simulink model "power_SVPWM_3Level"  (R2022a)
settings: Solver=FixedStepDiscrete  StartTime=0.0  StopTime=0.35  RelTol=1e-4  EnableMultiTasking=on
PreLoadFcn:
  | Ts=5e-6;          % Sample time (s)
StartFcn:
  | tic
StopFcn:
  | toc
undefined symbols (not defined in the file): D1, Delta, Lstat
libraries: spsSeriesRLCBranchLib x9, spsThreePhaseVIMeasurementLib x3, spsVoltageMeasurementLib x2, spsThreePhaseSourceLib x1, spsCurrentMeasurementLib x1, spsDCVoltageSourceLib x1, spsPower3phInstantaneousLib x1, spsSVPWMGenerator3LevelLib x1, spsIdealSwitchLib x1, spsThreeLevelNPCConverterLib x1, spsThreePhaseTransformerTwoWindingsLib x1, spspowerguiLib x1
settings Model: Creator=The MathWorks, Inc.  LastModifiedBy=jicai
settings SolverCC: AlgebraicLoopSolver=TrustRegion
settings DataIOCC: SaveFormat=Array  SaveOutput=off  SignalLogging=off  DSMLogging=off  SaveTime=off  ReturnWorkspaceOutputs=off
settings OptimizationCC: ExpressionDepthLimit=2147483647  LifeSpan=inf
settings DebuggingCC: UnderspecifiedInitializationDetection=Classic  MergeDetectMultiDrivingBlocksExec=none  SolverPrmCheckMsg=warning  SingleTaskRateTransMsg=warning  UnconnectedInputMsg=warning  UnconnectedOutputMsg=warning  UnconnectedLineMsg=warning  StateNameClashWarn=warning  SFUnexpectedBacktrackingDiag=warning  SFNoUnconditionalDefaultTransitionDiag=warning  SFExecutionAtInitializationDiag=none  SFMachineParentedDataDiag=warning  ArithmeticOperatorsInVariantConditions=warning
settings HardwareCC: ProdBitPerPointer=32  ProdBitPerSizeT=32  ProdBitPerPtrDiffT=32  ProdLargestAtomicFloat=None  ProdIntDivRoundTo=Undefined  ProdEndianess=Unspecified  ProdWordSize=32  ProdHWDeviceType=32-bit Generic
settings ModelReferenceCC: PropagateSignalLabelsOutOfModel=off
settings SFSimCC: SimUseLocalCustomCode=off  CustomCodeUndefinedFunction=UseInterfaceOnly
settings RTWCC: RTWUseLocalCustomCode=off
settings CodeAppCC: StateflowObjectComments=on
settings GRTTargetCC: TargetLangStandard=C89/C90 (ANSI)
settings ConfigComp: CovMetricSettings=dw  CovSaveCumulativeToWorkspaceVar=on  CovSaveSingleToWorkspaceVar=on  CovExternalEMLEnable=off
settings SimscapeCC: SimscapeNormalizeSystem=off

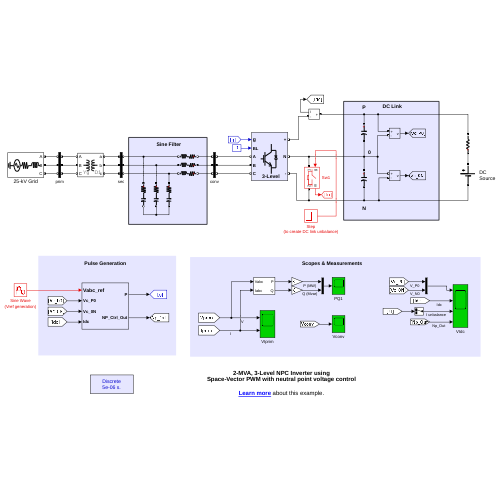
[thumbnail: Simulink's stored preview of the top-level diagram]
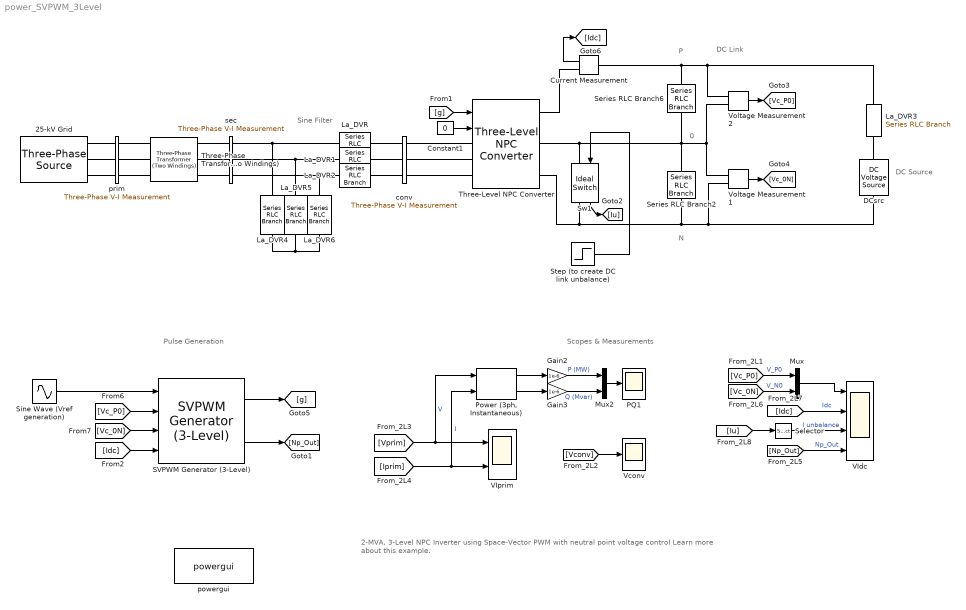
== system power_SVPWM_3Level ==
  note: DC
      | Source
  note: Scopes & Measurements
  note: 0
  note: 2-MVA, 3-Level NPC Inverter using
      | Space-Vector PWM with neutral point voltage control
      |
      | Learn more about this example.
  note: P
  note: N
  note: Sine Filter
  note: DC Link
  note: Pulse Generation
  25-kV Grid : spsThreePhaseSourceLib/Three-Phase Source  InternalConnection=Yg  VoltagePhases=off  Voltage=25e3  PhaseAngle=0  Voltage_phases=[25e3 25e3 25e3]/sqrt(3)  PhaseAngles_phases=[0 -120 +120]  Frequency=60  NonIdealSource=on  SpecifyImpedance=on  Resistance=0.8929  Inductance=16.58e-3  ShortCircuitLevel=200e6  BaseVoltage=25e3  XRratio=7  BusType=swing  Pref=10e3  Qref=0  Prefabc=[10e3, 10e3, 10e3]  Qrefabc=[0, 0, 0]  Qmin=-inf  Qmax=inf
  Constant1 : Constant  Value=0
  Current Measurement : spsCurrentMeasurementLib/Current Measurement  PhasorSimulation=off  OutputType=Complex  PSBequivalent=0
  DCsrc : spsDCVoltageSourceLib/DC Voltage Source  Amplitude=2400  Measurements=None
  Gain2 : Gain  Gain=1e-6
  Gain3 : Gain  Gain=1e-6
  La_DVR : spsSeriesRLCBranchLib/Series RLC Branch  LConnTagsString=__new0  RConnTagsString=__new0  BranchType=RL  Resistance=5e-3  Inductance=500e-6  SetiL0=off  InitialCurrent=0  Capacitance=1.0  Setx0=off  InitialVoltage=0  Measurements=None
  La_DVR1 : spsSeriesRLCBranchLib/Series RLC Branch  LConnTagsString=__new0  RConnTagsString=__new0  BranchType=RL  Resistance=5e-3  Inductance=500e-6  SetiL0=off  InitialCurrent=0  Capacitance=1.0  Setx0=off  InitialVoltage=0  Measurements=None
  La_DVR2 : spsSeriesRLCBranchLib/Series RLC Branch  LConnTagsString=__new0  RConnTagsString=__new0  BranchType=RL  Resistance=5e-3  Inductance=500e-6  SetiL0=off  InitialCurrent=0  Capacitance=1.0  Setx0=off  InitialVoltage=0  Measurements=None
  La_DVR3 : spsSeriesRLCBranchLib/Series RLC Branch  LConnTagsString=__new0  RConnTagsString=__new0  BranchType=R  Resistance=1e-3  Inductance=Lstat  SetiL0=off  InitialCurrent=0  Capacitance=1.0  Setx0=off  InitialVoltage=0  Measurements=None
  La_DVR4 : spsSeriesRLCBranchLib/Series RLC Branch  LConnTagsString=__new0  RConnTagsString=__new0  BranchType=RC  Resistance=1  Inductance=1  SetiL0=off  InitialCurrent=0  Capacitance=50e-6  Setx0=off  InitialVoltage=0  Measurements=None
  La_DVR5 : spsSeriesRLCBranchLib/Series RLC Branch  LConnTagsString=__new0  RConnTagsString=__new0  BranchType=RC  Resistance=1  Inductance=1  SetiL0=off  InitialCurrent=0  Capacitance=50e-6  Setx0=off  InitialVoltage=0  Measurements=None
  La_DVR6 : spsSeriesRLCBranchLib/Series RLC Branch  LConnTagsString=__new0  RConnTagsString=__new0  BranchType=RC  Resistance=1  Inductance=1  SetiL0=off  InitialCurrent=0  Capacitance=50e-6  Setx0=off  InitialVoltage=0  Measurements=None
  Mux : Mux  Inputs=2
  Mux2 : Mux  Inputs=2
  PQ1 : Scope
  "Power (3ph, Instantaneous)" : spsPower3phInstantaneousLib/Power (3ph, Instantaneous)
  SVPWM Generator (3-Level) : spsSVPWMGenerator3LevelLib/SVPWM Generator (3-Level)  InputType=Three-phase signals  Kp=0.04  fn=30  Fsw=1620  ParVref=[0.8 -30 60]  Ts=Ts
      settings: SourceProductBaseCode=PS
  Selector : Selector  InputPortWidth=2  IndexOptions=Index vector (dialog)  Indices=1  OutputSizes=1
  Series RLC Branch2 : spsSeriesRLCBranchLib/Series RLC Branch  LConnTagsString=__new0  RConnTagsString=__new0  BranchType=C  Resistance=1  Inductance=1e-3  SetiL0=off  InitialCurrent=0  Capacitance=15e-3  Setx0=on  InitialVoltage=1200  Measurements=None
  Series RLC Branch6 : spsSeriesRLCBranchLib/Series RLC Branch  LConnTagsString=__new0  RConnTagsString=__new0  BranchType=C  Resistance=1  Inductance=1e-3  SetiL0=off  InitialCurrent=0  Capacitance=15e-3  Setx0=on  InitialVoltage=1200  Measurements=None
  Sine Wave (Vref generation) : Sin  Amplitude=0.94  Frequency=2*pi*60  Phase=[0, -2*pi/3, 2*pi/3] -18*pi/180  SampleTime=Ts
  Step (to create DC link unbalance) : Step  Time=0.2  SampleTime=Ts
  Sw1 : spsIdealSwitchLib/Ideal Switch  Ron=100  Lon=0  IC=0  Rs=1e6  Cs=inf  Measurements=on
  Three-Level NPC Converter : spsThreeLevelNPCConverterLib/Three-Level NPC Converter  ModelType=Switching devices  Ron=1e-3  Rs=1e6  Cs=inf  Vforward=[0,0]  Ron_Diode=1e-3  Rs_Diode=1e6  Cs_Diode=inf  Vf_Diode=1e-3  Rs_CurrentSource=inf  Ron_ACsource=1e-3
      settings: SourceProductBaseCode=PS
  Three-Phase Transformer (Two Windings) : spsThreePhaseTransformerTwoWindingsLib/Three-Phase Transformer (Two Windings)  Winding1Connection=Yg  Winding2Connection=Delta (D1)  CoreType=Three single-phase transformers  SetSaturation=off  Hysteresis=off  DataFile='hysteresis'  SetInitialFlux=off  Measurements=None  UNITS=pu  NominalPower=[2e6, 60 ]  Winding1=[ 25e3, 0.0015, 0.03]  Winding2=[ 1.5e3, 0.0015, 0.03]  Rm=200  Lm=200  L0=0.5  Saturation=[ 0,0 ; 0.0024,1.2 ; 1.0,1.52 ]  InitialFluxes=[ 0.8 , -0.8 , 0.7 ]  BreakLoop=off  DiscreteSolver=Trapezoidal iterative  DataType=off  TransfoNumber=1
  VIdc : Scope  NumInputPorts=4
  VIprim : Scope  NumInputPorts=2
  Vconv : Scope
  Voltage Measurement1 : spsVoltageMeasurementLib/Voltage Measurement  PhasorSimulation=off  OutputType=Complex  PSBequivalent=0
  Voltage Measurement2 : spsVoltageMeasurementLib/Voltage Measurement  PhasorSimulation=off  OutputType=Complex  PSBequivalent=0
  conv : spsThreePhaseVIMeasurementLib/Three-Phase V-I Measurement  VoltageMeasurement=phase-to-phase  SetLabelV=on  LabelV=Vconv  Vpu=off  VpuLL=off  CurrentMeasurement=no  SetLabelI=on  LabelI=Isec  Ipu=off  Pbase=100e6  Vbase=500e3  OutputType=Complex  PhasorSimulation=off  PSBequivalent=0
  powergui : spspowerguiLib/powergui  Priority=1  SimulationMode=Discrete  SampleTime=Ts  frequency=60  Iterations=50  frequencyindice=0  Pbase=100e6  ErrMax=1e-4  UnitsV=kV  UnitsW=MW  buscounter=0  FunctionMessages=off  echomessages=off  EnableUseOfTLC=off  CurrentSourceSwitches=off  DisableSnubberDevices=on  DisableRonSwitches=off  DisableVfSwitches=off  DisplayEquations=off  AutomaticDiscreteSolvers=off  SolverType=Tustin/Backward Euler (TBE)  Interpol=off  ExternalGateDelay=off  methode=off  Ts=10  x0status=blocks  SPID=on  SwTol=0  HookPort=off  NonlinearTolerance=1e-4  nMaxIteration=100  ContinueOnMaxIteration=off  RestoreLinks=warning  ResistiveCurrentMeasurement=off  Frange=[0:2:500]  Ylog=off  Xlog=on  ShowGrid=off  save=off  variable=ZData  structure=Vconv  ZoomFFT=off  StartTime=0.33  cycles=1  DisplayStyle=1  fundamental=60  FreqAxis=off  MaxFrequency=6000  frequencyindicesteady=1  RmsSteady=1  display=off
  prim : spsThreePhaseVIMeasurementLib/Three-Phase V-I Measurement  VoltageMeasurement=phase-to-ground  SetLabelV=on  LabelV=Vprim  Vpu=off  VpuLL=off  CurrentMeasurement=yes  SetLabelI=on  LabelI=Iprim  Ipu=off  Pbase=100e6  Vbase=500e3  OutputType=Complex  PhasorSimulation=off  PSBequivalent=0
  sec : spsThreePhaseVIMeasurementLib/Three-Phase V-I Measurement  VoltageMeasurement=no  SetLabelV=on  LabelV=Vsec  Vpu=off  VpuLL=off  CurrentMeasurement=no  SetLabelI=on  LabelI=Isec  Ipu=off  Pbase=100e6  Vbase=500e3  OutputType=Complex  PhasorSimulation=off  PSBequivalent=0
  wires:
  Constant1/1 -> Three-Level NPC Converter/2
  [g] -> Three-Level NPC Converter/1
  Current Measurement/1 -> [Idc]
  Voltage Measurement2/1 -> [Vc_P0]
  Voltage Measurement1/1 -> [Vc_0N]
  Step (to create DC link unbalance)/1 -> Sw1/1
  [Vprim] -> VIprim/1, "Power (3ph, Instantaneous)"/1  "V"
  [Iprim] -> VIprim/2, "Power (3ph, Instantaneous)"/2  "I"
  [Vc_P0] -> Mux/1  "V_P0"
  [Vc_0N] -> Mux/2  "V_N0"
  Mux/1 -> VIdc/1
  [Idc] -> VIdc/2  "Idc"
  SVPWM Generator (3-Level)/2 -> [Np_Out]
  SVPWM Generator (3-Level)/1 -> [g]
  [Vc_P0] -> SVPWM Generator (3-Level)/2
  [Vc_0N] -> SVPWM Generator (3-Level)/3
  [Idc] -> SVPWM Generator (3-Level)/4
  Mux2/1 -> PQ1/1
  Gain2/1 -> Mux2/1  "P (MW)"
  Gain3/1 -> Mux2/2  "Q (Mvar)"
  "Power (3ph, Instantaneous)"/1 -> Gain2/1
  "Power (3ph, Instantaneous)"/2 -> Gain3/1
  Sine Wave (Vref generation)/1 -> SVPWM Generator (3-Level)/1
  Sw1/1 -> [Iu]
  [Iu] -> Selector/1
  [Np_Out] -> VIdc/4  "Np_Out"
  Selector/1 -> VIdc/3  "I unbalance"
  [Vconv] -> Vconv/1
  connections:
  Series RLC Branch6/LConn1 -- La_DVR3/RConn1 -- Voltage Measurement2/LConn1 -- Current Measurement/LConn1
  25-kV Grid/RConn2 -- prim/RConn2
  25-kV Grid/RConn3 -- prim/RConn3
  sec/LConn1 -- La_DVR4/LConn1 -- La_DVR/RConn1
  sec/LConn3 -- La_DVR2/RConn1 -- La_DVR6/LConn1
  sec/LConn2 -- La_DVR1/RConn1 -- La_DVR5/LConn1
  25-kV Grid/RConn1 -- prim/RConn1
  prim/LConn3 -- Three-Phase Transformer (Two Windings)/LConn3
  Three-Phase Transformer (Two Windings)/RConn1 -- sec/RConn1
  Three-Level NPC Converter/RConn1 -- Current Measurement/RConn1
  prim/LConn1 -- Three-Phase Transformer (Two Windings)/LConn1
  Three-Phase Transformer (Two Windings)/RConn2 -- sec/RConn2
  prim/LConn2 -- Three-Phase Transformer (Two Windings)/LConn2
  Three-Phase Transformer (Two Windings)/RConn3 -- sec/RConn3
  Series RLC Branch2/LConn1 -- Three-Level NPC Converter/RConn2 -- Sw1/LConn1 -- Voltage Measurement2/LConn2 -- Voltage Measurement1/LConn1 -- Series RLC Branch6/RConn1
  Three-Level NPC Converter/RConn3 -- DCsrc/LConn1 -- Voltage Measurement1/LConn2 -- Series RLC Branch2/RConn1 -- Sw1/RConn1
  La_DVR3/LConn1 -- DCsrc/RConn1
  La_DVR4/RConn1 -- La_DVR6/RConn1 -- La_DVR5/RConn1
  conv/RConn1 -- La_DVR/LConn1
  La_DVR1/LConn1 -- conv/RConn2
  La_DVR2/LConn1 -- conv/RConn3
  conv/LConn1 -- Three-Level NPC Converter/LConn1
  conv/LConn2 -- Three-Level NPC Converter/LConn2
  conv/LConn3 -- Three-Level NPC Converter/LConn3
